simulink model "uz_flux_prediction"  (R2023b)
settings: Solver=FixedStepDiscrete  StartTime=0.0  StopTime=0.1  RelTol=1e-3  EnableMultiTasking=on
PreLoadFcn:
  | uz_setCodegenPaths
model workspace (MATLAB code in the model file):
  | cmdLim = Simulink.Parameter;
  | cmdLim.Value = 15;
  | cmdLim.Description = 'Limit for controlling the maximum surface command angle.';
  | cmdLim.Min = 0;
  | cmdLim.Max = 90;
  | cmdLim.DocUnits = 'deg';
  | 
  | dispGain = Simulink.Parameter;
  | dispGain.Value = 0.75;
  | dispGain.Description = 'Gain applied to the displacement error.';
  | dispGain.Min = 0;
  | dispGain.Max = [];
  | dispGain.DocUnits = 'deg/sec/deg';
  | 
  | dispLim = Simulink.Parameter;
  | dispLim.Value = 30;
  | dispLim.Description = 'Limit for controlling the maximum commanded angle.';
  | dispLim.Min = 0;
  | dispLim.Max = 180;
  | dispLim.DocUnits = 'deg';
  | 
  | intGain = Simulink.Parameter;
  | intGain.Value = 0.5;
  | intGain.Description = 'Gain applied to the integral error.';
  | intGain.Min = 0;
  | intGain.Max = [];
  | intGain.DocUnits = 'deg/sec/deg/sec';
  | 
  | intLim = Simulink.Parameter;
  | intLim.Value = 5;
  | intLim.Description = 'Limit for controlling the maximum commanded angle.';
  | intLim.Min = 0;
  | intLim.Max = 90;
  | intLim.DocUnits = 'deg';
  | 
  | rateGain = Simulink.Parameter;
  | rateGain.Value = 2;
  | rateGain.Description = 'Gain applied to the rate error.';
  | rateGain.Min = 0;
  | rateGain.Max = [];
  | rateGain.DocUnits = 'deg/deg/sec';
  | 
  | rateLim = Simulink.Parameter;
  | rateLim.Value = 6;
  | rateLim.Description = 'Limit for controlling the maximum commanded angle.';
  | rateLim.Min = 0;
  | rateLim.Max = 180;
  | rateLim.DocUnits = 'deg/sec';
  | 
  | hdgGain = Simulink.Parameter;
  | hdgGain.Value = 0.015;
undefined symbols (not defined in the file or in its folder): ts_regler
settings Model: RequirementInfo={} %GIDa_fe9045fd_0412_4b6e_8206_617cc20e6fde  FPTRunName=Active  Creator=ts  LastModifiedBy=Philipp
settings SolverCC: AlgebraicLoopSolver=TrustRegion  PositivePriorityOrder=on  AutoInsertRateTranBlk=on
settings DataIOCC: SaveOutput=off  SignalLogging=off  DSMLogging=off  SaveTime=off
settings OptimizationCC: DefaultParameterBehavior=Inlined  UseDivisionForNetSlopeComputation=on  GainParamInheritBuiltInType=on  UseFloatMulNetSlope=on  UseSpecifiedMinMax=on  InlineInvariantSignals=on  PassReuseOutputArgsAs=Individual arguments  NoFixptDivByZeroProtection=on  EfficientFloat2IntCast=on  LifeSpan=1  MaxStackSize=64  OptimizeBlockOrder=speed  DifferentSizesBufferReuse=on  EfficientTunableParamExpr=on
settings DebuggingCC: UnconnectedInputMsg=warning  UnconnectedOutputMsg=warning  UnconnectedLineMsg=warning  AllowSymbolicDim=off  SFUnexpectedBacktrackingDiag=warning  SFNoUnconditionalDefaultTransitionDiag=warning  SFExecutionAtInitializationDiag=none  ArithmeticOperatorsInVariantConditions=warning
settings HardwareCC: ProdBitPerPointer=32  ProdBitPerSizeT=32  ProdBitPerPtrDiffT=32  ProdLargestAtomicInteger=Long  ProdLargestAtomicFloat=Double  ProdWordSize=32  ProdLongLongMode=on  ProdHWDeviceType=ARM Compatible->ARM Cortex-R  HardwareBoardFeatureSet=SoCBlockset
settings ModelReferenceCC: EnableRefExpFcnMdlSchedulingChecks=on
settings SFSimCC: MATLABDynamicMemAlloc=off
settings RTWCC: Description=Embedded Coder  SystemTargetFile=ert.tlc  GenCodeOnly=on  TemplateMakefile=ert_default_tmf  GenerateReport=on  BuildConfiguration=Faster Runs  IncludeHyperlinkInReport=on  GenerateCodeMetricsReport=on  CheckMdlBeforeBuild=Warning  DLArmComputeVersion=19.05
settings CodeAppCC: ForceParamTrailComments=on  IgnoreCustomStorageClasses=off  OperatorAnnotations=on  SimulinkDataObjDesc=on  SFDataObjDesc=on  MATLABFcnDesc=on  CustomSymbolStrGlobalVar=rt$N$M  CustomSymbolStrType=$N$M  CustomSymbolStrFcn=$N$M$F  CustomSymbolStrMacro=$N$M  InsertBlockDesc=on  StateflowObjectComments=on  MATLABSourceComments=on  EnableCustomComments=on  ReqsInCode=on
settings ERTTargetCC: TargetLangStandard=C99 (ISO)  CodeReplacementLibrary=GNU C99 extensions  MultiwordLength=2048  IncludeMdlTerminateFcn=off  CombineSignalStateStructs=on  SuppressErrorStatus=on  IncludeFileDelimiter=UseQuote  SupportAbsoluteTime=off  CodeInterfacePackaging=Reusable function  SupportNonFinite=off  RemoveResetFunc=off  InlinedParameterPlacement=NonHierarchical  MultiInstanceErrorCode=Warning  RootIOFormat=Part of model data structure  ERTCustomFileTemplate=example_file_process.tlc  GlobalDataDefinition=InSourceFile  GlobalDataReference=InSourceFile  ERTFilePackagingFormat=CompactWithDataFile
settings ConfigComp: CovScope=ReferencedModels  CovSaveName=covdata_rollAP  CovMetricSettings=dcmtrwe  CovHTMLOptions=-sRT=1 -aTS=1 -bRG=1 -bTC=1 -hTR=1 -nFC=0 -scm=1 -bcm=1 -xEv=0  CovSaveCumulativeToWorkspaceVar=on  CovSaveSingleToWorkspaceVar=on  CovCumulativeVarName=covCumulativeData_rollAP  CovReportOnPause=off  CovExternalEMLEnable=off  CovSFcnEnable=off

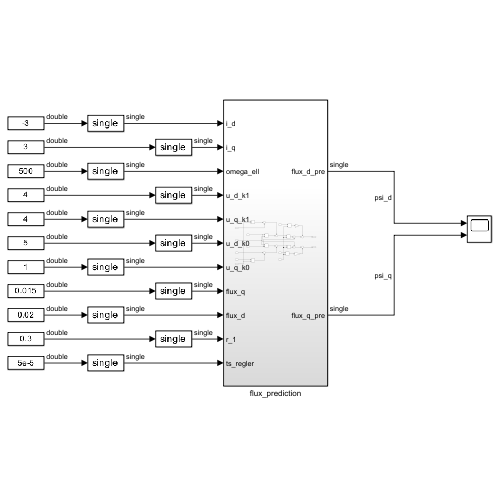
[thumbnail: Simulink's stored preview of the top-level diagram]
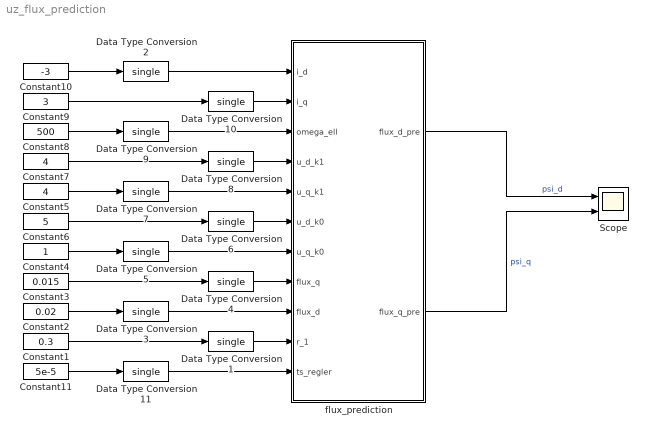
== system uz_flux_prediction ==
  Constant1 : Constant  Value=0.3
  Constant10 : Constant  Value=-3
  Constant11 : Constant  Value=5e-5
  Constant2 : Constant  Value=0.02
  Constant3 : Constant  Value=0.015
  Constant4 : Constant
  Constant5 : Constant  Value=4
  Constant6 : Constant  Value=5
  Constant7 : Constant  Value=4
  Constant8 : Constant  Value=500
  Constant9 : Constant  Value=3
  Data Type Conversion{1..11} (11 alike) : DataTypeConversion  OutDataTypeStr=single  SaturateOnIntegerOverflow=off  RndMeth=Floor
  Scope : Scope  NumInputPorts=2
  flux_prediction : Subsystem
  wires:
  flux_prediction/1(flux_d_pre) -> Scope/1  "psi_d"
  Constant10/1 -> Data Type Conversion2/1
  Data Type Conversion2/1 -> flux_prediction/1(i_d)
  flux_prediction/2(flux_q_pre) -> Scope/2  "psi_q"
  Constant3/1 -> Data Type Conversion4/1
  Data Type Conversion3/1 -> flux_prediction/9(flux_d)
  Constant2/1 -> Data Type Conversion3/1
  Data Type Conversion4/1 -> flux_prediction/8(flux_q)
  Constant6/1 -> Data Type Conversion6/1
  Constant4/1 -> Data Type Conversion5/1
  Data Type Conversion5/1 -> flux_prediction/7(u_q_k0)
  Data Type Conversion6/1 -> flux_prediction/6(u_d_k0)
  Constant9/1 -> Data Type Conversion10/1
  Constant8/1 -> Data Type Conversion9/1
  Data Type Conversion9/1 -> flux_prediction/3(omega_ell)
  Constant7/1 -> Data Type Conversion8/1
  Constant5/1 -> Data Type Conversion7/1
  Data Type Conversion8/1 -> flux_prediction/4(u_d_k1)
  Data Type Conversion7/1 -> flux_prediction/5(u_q_k1)
  Data Type Conversion10/1 -> flux_prediction/2(i_q)
  Constant1/1 -> Data Type Conversion1/1
  Data Type Conversion1/1 -> flux_prediction/10(r_1)
  Constant11/1 -> Data Type Conversion11/1
  Data Type Conversion11/1 -> flux_prediction/11(ts_regler)

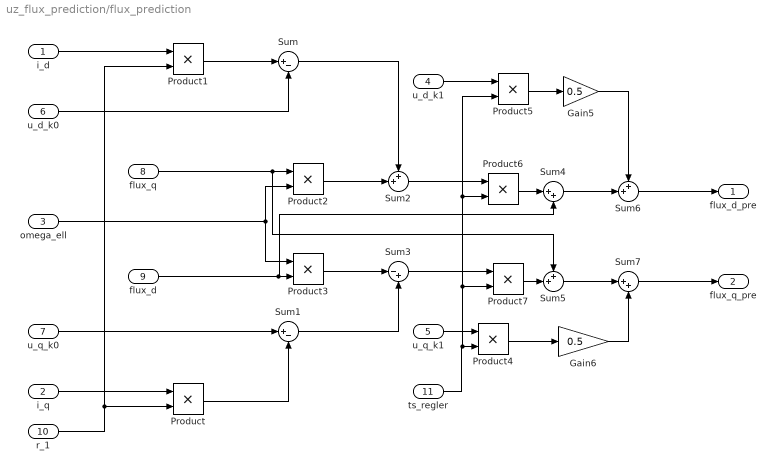
== system uz_flux_prediction/flux_prediction ==
  i_d : Inport
  i_q : Inport  Port=2
  omega_ell : Inport  Port=3
  u_d_k1 : Inport  Port=4  SampleTime=ts_regler
  u_q_k1 : Inport  Port=5
  u_d_k0 : Inport  Port=6
  u_q_k0 : Inport  Port=7
  flux_q : Inport  Port=8
  flux_d : Inport  Port=9
  r_1 : Inport  Port=10
  ts_regler : Inport  Port=11
  Gain5 : Gain  Gain=0.5  OutDataTypeStr=Inherit: Same as input
  Gain6 : Gain  Gain=0.5
  Product{,1..7} (8 alike) : Product
  Sum : Sum  Inputs=|+-
  Sum1 : Sum  Inputs=|+-
  Sum2 : Sum  Inputs=++|
  Sum3 : Sum  Inputs=|-+
  Sum4 : Sum  Inputs=|++
  Sum5 : Sum  Inputs=++|
  Sum6 : Sum  Inputs=++|
  Sum7 : Sum  Inputs=|++
  flux_d_pre : Outport
  flux_q_pre : Outport  Port=2
  wires:
  flux_q/1 -> Product2/1, Sum5/1
  flux_d/1 -> Product3/2, Sum4/2
  omega_ell/1 -> Product3/1, Product2/2
  u_d_k0/1 -> Sum/2
  Product1/1 -> Sum/1
  u_q_k0/1 -> Sum1/1
  Product/1 -> Sum1/2
  Product3/1 -> Sum3/1
  Product2/1 -> Sum2/2
  Sum/1 -> Sum2/1
  Sum1/1 -> Sum3/2
  Sum3/1 -> Product7/1
  Sum2/1 -> Product6/1
  Product6/1 -> Sum4/1
  Product7/1 -> Sum5/2
  Sum4/1 -> Sum6/2
  Gain5/1 -> Sum6/1
  Sum5/1 -> Sum7/1
  Gain6/1 -> Sum7/2
  i_d/1 -> Product1/1
  i_q/1 -> Product/1
  Sum7/1 -> flux_q_pre/1
  Sum6/1 -> flux_d_pre/1
  r_1/1 -> Product/2, Product1/2
  Product4/1 -> Gain6/1
  u_q_k1/1 -> Product4/1
  ts_regler/1 -> Product7/2, Product5/2, Product6/2, Product4/2
  Product5/1 -> Gain5/1
  u_d_k1/1 -> Product5/1
